simulink model "KFgain"  (Simulink 7.0)
settings: Solver=FixedStepDiscrete  StartTime=0.0  StopTime=10.0  RelTol=1e-3
values from neighbouring files (symbols this model uses):
  A1 = A    (= 0)    [feedbackviewKF.m]
  C1 = C    (= 1)    [feedbackviewKF.m]
  P1 = 10*eye(4)    [feedbackviewKF.m]
  Q1 = Q    (= 4)    [feedbackviewKF.m]
  R1 = R    (= 1)    [feedbackviewKF.m]
settings Model: Creator=fo1521  LastModifiedBy=fo1521

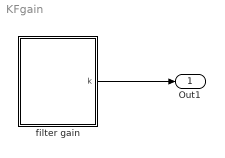
== system KFgain ==
  filter gain : Subsystem  mask{P0=P1, A=A1, C=C1, Q=Q1, R=R1}
      mask Display: disp(sprintf('Kalman\n Filter\n Gain'))
  Out1 : Outport  OutDataType=sfix(16)  OutScaling=2^0
  wires:
  filter gain/1(k) -> Out1/1

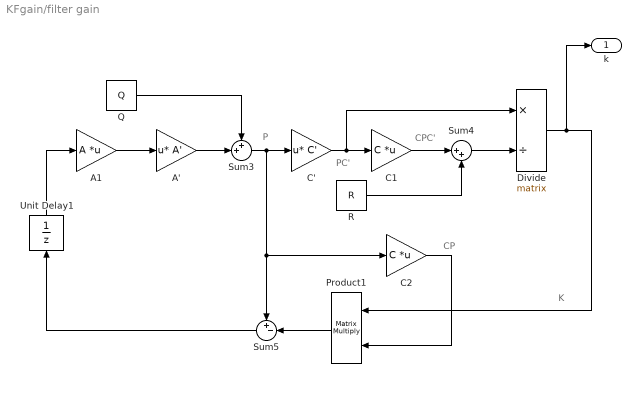
== system KFgain/filter gain ==
  note: P
  note: PC'
  note: CPC'
  note: K
  note: CP
  A' : Gain  Gain=A'  Multiplication=Matrix(u*K)  ParameterDataType=sfix(16)  ParameterScaling=2^0  OutDataType=sfix(16)  OutScaling=2^0
  A1 : Gain  Gain=A  Multiplication=Matrix(K*u)  ParameterDataType=sfix(16)  ParameterScaling=2^0  OutDataType=sfix(16)  OutScaling=2^0
  C' : Gain  Gain=C'  Multiplication=Matrix(u*K)  ParameterDataType=sfix(16)  ParameterScaling=2^0  OutDataType=sfix(16)  OutScaling=2^0
  C1 : Gain  Gain=C  Multiplication=Matrix(K*u)  ParameterDataType=sfix(16)  ParameterScaling=2^0  OutDataType=sfix(16)  OutScaling=2^0
  C2 : Gain  Gain=C  Multiplication=Matrix(K*u)  ParameterDataType=sfix(16)  ParameterScaling=2^0  OutDataType=sfix(16)  OutScaling=2^0
  Divide : Product  Inputs=*/  Multiplication=Matrix(*)  OutDataType=sfix(16)  OutScaling=2^-10
  Product1 : Product  Orientation=left  Multiplication=Matrix(*)  OutDataType=sfix(16)  OutScaling=2^0  RndMeth=Zero
  Q : Constant  Value=Q  OutDataType=sfix(16)  OutScaling=2^0
  R : Constant  Value=R  OutDataType=sfix(16)  OutScaling=2^0
  Sum3 : Sum  Inputs=++|  OutDataType=sfix(16)  OutScaling=2^0
  Sum4 : Sum  Inputs=|++  OutDataType=sfix(16)  OutScaling=2^0
  Sum5 : Sum  Orientation=left  Inputs=+-|  OutDataType=sfix(16)  OutScaling=2^0
  Unit Delay1 : UnitDelay  Orientation=up  X0=P0
  k : Outport  OutDataType=sfix(16)  OutScaling=2^0
  wires:
  A1/1 -> A'/1
  A'/1 -> Sum3/2
  Q/1 -> Sum3/1
  Sum3/1 -> C'/1, Sum5/1, C2/1
  C'/1 -> C1/1, Divide/1
  Divide/1 -> Product1/1, k/1
  Product1/1 -> Sum5/2
  C1/1 -> Sum4/1
  R/1 -> Sum4/2
  Sum4/1 -> Divide/2
  Unit Delay1/1 -> A1/1
  Sum5/1 -> Unit Delay1/1
  C2/1 -> Product1/2
